simulink model "PubIfDecisionTOS_MDL"  (R2020b)
settings: configuration reference "DspaceConfig" (kept outside this file)
PostLoadFcn:
  | if any(exist('dsrtsu_mdlpostloadfcn', 'file') ~= 0), dsrtsu_mdlpostloadfcn('Execute', bdroot); end
InitFcn:
  | , if any(exist('dsmpb_private', 'file') ~= 0), dsmpb_private('dsmpb_mdlclblib', 'Init', bdroot); end,
undefined symbols (not defined in the file or in its folder): C_TOS_ACCEgoRAxletoFbumplength_m, C_TOS_ACCTargetFront_Flag, C_TOS_AEBJAPedObjDxThre_Val, C_TOS_AEBJAPedObjDyThre_Val, C_TOS_AEBJATargetSize_Val, C_TOS_AEBJAVehObjDxThre_Val, C_TOS_AEBJAVehObjDyThre_Val, C_TOS_AEBJuncPedTargetSize_Val, C_TOS_AEBLatObjDxThre_Val, C_TOS_AEBLatPedDyThre_Val, C_TOS_AEBLatTargetSize_Val, C_TOS_AEBLongTargetInEgoFront_Flag, C_TOS_axAbsGround_Parameter, C_TOS_CameraConfirmedFlag, C_TOS_CNsubjWidth, C_TOS_CurrentLaneCoreMinWidth_Val, C_TOS_CutInProb_Val_Zero, C_TOS_CutOutProb_Val_Zero, C_TOS_D2R_Val, C_TOS_DefaultValueObjectToCenterLine_dy, C_TOS_EgoCarWidth_Val, C_TOS_EgoDxRefPoint_m, C_TOS_EgoRAxletoFbumplength_m, C_TOS_HalfWidthVehicle_Con, C_TOS_HWA_CurrentLaneFlag, C_TOS_HWA_LeftLaneFlag, C_TOS_HWA_MovingDir_Vaild, C_TOS_HWA_MovState_Vaild, C_TOS_HWA_RightLaneFlag, C_TOS_LaneLineCourseErrorFront, C_TOS_LaneLineCourseErrorRear, C_TOS_MotorbikeDefaultWidth_m, C_TOS_NumberOfEffectiveTargets, C_TOS_Obj_Age_Val, C_TOS_Objdx_Constraint_Val, C_TOS_ObjectDefaultWidth_m, C_TOS_ObjInCurrentLane_Val, C_TOS_ObjInCurrentLaneValid, C_TOS_ObjInLeftLaneValid, C_TOS_ObjInRightLaneValid, C_TOS_ObjNotInCurrentLane_Val, C_TOS_ObjNotREElementType, C_TOS_ObjPredictDis_dy_ConstantVal_Zeros, C_TOS_ObjToCenterLine_ConstantVal_Zeros, C_TOS_OFMObjIDInvilad_Val, C_TOS_PIL_LatDisCons_Val_zero, C_TOS_PIL_ObjectCutInFlag_b, C_TOS_PIL_ObjectCutOutFlag_b, C_TOS_PIL_ObjLaneProb_al_Val, C_TOS_PP_ObjFusType_FC_Confirm_b, C_TOS_PP_ObjFusType_FC_FR_Confirm_b, C_TOS_PP_ObjFusType_FR_Confirm_b, C_TOS_RE_80BoolDefault_Val, C_TOS_RE_80Single181Default_Val, C_TOS_RE_80Single255Default_Val, C_TOS_RE_80Uint8Default_Val, C_TOS_RE_D2R, C_TOS_RE_D_180_Val, C_TOS_RE_InvalidObjectID_Val, C_TOS_RE_InvalidTargetChainDir_Val ... (+142)
libraries: simulink x1650, TOS_LIB x361, canfdmsglib x14
(part 65 of 69)

== stateflow chart PubIfDecisionTOS_MDL/TOS_20201112/TOS_2012080320/TOS/AEB/TOS_AEBJunct1105/AEBJunctionTargetInfor/TOS_AEBJunct ==
  (default) -> (junction 1) : {i=uint8(1);}
  (junction 1) -> (junction 40) [order 1] : [i<=C_TOS_AEBJATargetSize_Val]
  (junction 42) -> (junction 1) : {i=i+uint8(1);}
  (junction 1) -> (junction 60) [order 2]
  (junction 40) -> (junction 42) : {
      | TOS_AEBJuncTargetBus(i).FusionType= uint8(0);
      | TOS_AEBJuncTargetBus(i).ObjectID= uint8(0);
      | TOS_AEBJuncTargetBus(i).ObjectType= uint8(0);
      | TOS_AEBJuncTargetBus(i).ObjectTypeCameraConfirmed= false;
      | TOS_AEBJuncTargetBus(i).ObjectLength=single(0);
      | TOS_AEBJuncTargetBus(i).ObjectWidth= single(0);
      | TOS_AEBJuncTargetBus(i).ObjectHight= single(0);
      | TOS_AEBJuncTargetBus(i).ObjectYawAngle= single(0);
      | TOS_AEBJuncTargetBus(i).ObjectAzimuthAngle= single(0);
      | TOS_AEBJuncTargetBus(i).ObjectMovingState= uint8(0);
      | TOS_AEBJuncTargetBus(i).ObjectMovingOrientation=uint8(0);
      | TOS_AEBJuncTargetBus(i).dxFisrtDetection= single(0);
      | TOS_AEBJuncTargetBus(i).dyFisrtDetection= single(0);
      | TOS_AEBJuncTargetBus(i).dx= single(0);
      | TOS_AEBJuncTargetBus(i).dy= single(0);
      | TOS_AEBJuncTargetBus(i).dz= single(0);
      | TOS_AEBJuncTargetBus(i).vx= single(0);
      | TOS_AEBJuncTargetBus(i).vy= single(0);
      | TOS_AEBJuncTargetBus(i).ax= single(0);
      | TOS_AEBJuncTargetBus(i).ay= single(0);
      | TOS_AEBJuncTargetBus(i).dxVariance= single(0);
      | TOS_AEBJuncTargetBus(i).dyVariance= single(0);
      | TOS_AEBJuncTargetBus(i).vxVariance= single(0);
      | TOS_AEBJuncTargetBus(i).vyVariance= single(0);
      | TOS_AEBJuncTargetBus(i).axVariance= single(0);
      | TOS_AEBJuncTargetBus(i).ayVariance= single(0);
      | TOS_AEBJuncTargetBus(i).ObjectLengthVar= single(0);
      | TOS_AEBJuncTargetBus(i).ObjectWidthVar= single(0);
      | TOS_AEBJuncTargetBus(i).ObjectYawAngleVar= single(0);
      | TOS_AEBJuncTargetBus(i).ObjectTypeProb= single(0);
      | TOS_AEBJuncTargetBus(i).ObjectMovingStateProb= single(0);
      | TOS_AEBJuncTargetBus(i).ObjectMovingOrientationProb= single(0);
      | TOS_AEBJuncTargetBus(i).ObjectExistProb= single(0);
      | TOS_AEBJuncTargetBus(i).ObjectIsObstacleProb= single(0);
      | TOS_AEBJuncTargetBus(i).ObjectRCS= single(0);
      | TOS_AEBJuncTargetBus(i).ObjectMeasurementStatus= single(0);
      | TOS_AEBJuncTargetBus(i).ObjectLifeCycle= uint16(0);
      | TOS_AEBJuncTargetBus(i).ObjUpdate= false;
      | }
  (junction 60) -> (junction 53) : {i=uint8(1);
      | j=uint8(1);}
  (junction 53) -> (junction 62) [order 1] : [i<=C_TOS_AEBJATargetSize_Val]
  (junction 66) -> (junction 53) : {i=i+uint8(1);}
  (junction 53) -> (junction 46) [order 2]
  (junction 62) -> (junction 64)
  (junction 64) -> (junction 3) [order 1] : [TOS_AEBJATargetIndex(i)~=uint8(0)]
  (junction 64) -> (junction 66) [order 2]
  (junction 3) -> (junction 5) : {
      | TargetIndex = TOS_AEBJATargetIndex(i);
      | TOS_AEBJuncTargetBus(j).FusionType=OFM_SignalVerification.Object_Fus_Type(TargetIndex);
      | TOS_AEBJuncTargetBus(j).ObjectID=OFM_SignalVerification.Object_ID(TargetIndex);
      | TOS_AEBJuncTargetBus(j).ObjectType=AEBJuncTargetObjectType(i);
      | TOS_AEBJuncTargetBus(j).ObjectTypeCameraConfirmed=TOS_AddAttributes.PP_CamareConfirmSignalProcessing(TargetIndex);
      | TOS_AEBJuncTargetBus(j).ObjectLength=OFM_SignalVerification.Object_Length(TargetIndex);
      | TOS_AEBJuncTargetBus(j).ObjectWidth=OFM_SignalVerification.Object_Width(TargetIndex);
      | TOS_AEBJuncTargetBus(j).ObjectHight=OFM_SignalVerification.Object_Hight(TargetIndex);
      | TOS_AEBJuncTargetBus(j).ObjectYawAngle=OFM_SignalVerification.Object_HeadingAngle(TargetIndex);
      | TOS_AEBJuncTargetBus(j).ObjectAzimuthAngle=OFM_SignalVerification.Object_YawAngle(TargetIndex);
      | TOS_AEBJuncTargetBus(j).ObjectMovingState=TOS_AddAttributes.PP_MovingState_AEB_SignalProcessing(TargetIndex);
      | TOS_AEBJuncTargetBus(j).ObjectMovingOrientation=TOS_AddAttributes.PP_ObjMovingDirSignalProcessing(TargetIndex);
      | TOS_AEBJuncTargetBus(j).dxFisrtDetection=TOS_AddAttributes.PP_ObjFirstDetect_Dx(TargetIndex);
      | TOS_AEBJuncTargetBus(j).dyFisrtDetection=TOS_AddAttributes.PP_ObjFirstDetect_Dy(TargetIndex);
      | TOS_AEBJuncTargetBus(j).dx=OFM_SignalVerification.Object_DX(TargetIndex);
      | TOS_AEBJuncTargetBus(j).dy=OFM_SignalVerification.Object_DY(TargetIndex);
      | TOS_AEBJuncTargetBus(j).dz= single(0);
      | TOS_AEBJuncTargetBus(j).vx=OFM_SignalVerification.Object_VX(TargetIndex);
      | TOS_AEBJuncTargetBus(j).vy=OFM_SignalVerification.Object_VY(TargetIndex);
      | TOS_AEBJuncTargetBus(j).ax=OFM_SignalVerification.Object_AX(TargetIndex);
      | TOS_AEBJuncTargetBus(j).ay=OFM_SignalVerification.Object_AY(TargetIndex);
      | TOS_AEBJuncTargetBus(j).dxVariance=OFM_SignalVerification.Object_Std_DX(TargetIndex);
      | TOS_AEBJuncTargetBus(j).dyVariance=OFM_SignalVerification.Object_Std_DY(TargetIndex);
      | TOS_AEBJuncTargetBus(j).vxVariance=OFM_SignalVerification.Object_Std_VX(TargetIndex);
      | TOS_AEBJuncTargetBus(j).vyVariance=OFM_SignalVerification.Object_Std_VY(TargetIndex);
      | TOS_AEBJuncTargetBus(j).axVariance=OFM_SignalVerification.Object_Std_AX(TargetIndex);
      | TOS_AEBJuncTargetBus(j).ayVariance=OFM_SignalVerification.Object_Std_AY(TargetIndex);
      | TOS_AEBJuncTargetBus(j).ObjectLengthVar=OFM_SignalVerification.Object_Std_Length(TargetIndex);
      | TOS_AEBJuncTargetBus(j).ObjectWidthVar=OFM_SignalVerification.Object_Std_Width(TargetIndex);
      | TOS_AEBJuncTargetBus(j).ObjectYawAngleVar=OFM_SignalVerification.Object_Std_HeadingAngle(TargetIndex);
      | TOS_AEBJuncTargetBus(j).ObjectTypeProb=OFM_SignalVerification.Object_Type_Prob(TargetIndex);
      | TOS_AEBJuncTargetBus(j).ObjectMovingStateProb= single(0);
      | TOS_AEBJuncTargetBus(j).ObjectMovingOrientationProb= single(0);
      | TOS_AEBJuncTargetBus(j).ObjectExistProb=OFM_SignalVerification.Object_ExistProb(TargetIndex);
      | TOS_AEBJuncTargetBus(j).ObjectIsObstacleProb=OFM_SignalVerification.Object_ObstacleProb(TargetIndex);
      | TOS_AEBJuncTargetBus(j).ObjectRCS= single(0);
      | TOS_AEBJuncTargetBus(j).ObjectMeasurementStatus= single(0);
      | TOS_AEBJuncTargetBus(j).ObjectLifeCycle=OFM_SignalVerification.Object_Age(TargetIndex);
      | TOS_AEBJuncTargetBus(j).ObjUpdate= false;
      | j=j+uint8(1);
      | }
  (junction 5) -> (junction 66)
  data: TOS_AddAttributes input Bus: TOS_AddAttributes_BUS; OFM_SignalVerification input Bus: OFM_OBJ_BUS; AEBJuncTargetObjectType input uint8; TOS_AEBJATargetIndex input uint8; TOS_AEBJuncTargetBus output Bus: TOS_AEB_JAOBJ_BUS size=32 =0; C_TOS_AEBJATargetSize_Val parameter; TargetIndex local uint8 size=1; i local uint8 size=1; j local uint8 size=1

== matlab function PubIfDecisionTOS_MDL/TOS_20201112/TOS_2012080320/TOS/AEB/TOS_AEBJunct_20201208/AEBJuncTargetIndex/MATLAB Function ==
  data: Distance input; Object_Num input; ObjDisIndex output
function ObjDisIndex  = fcn(Distance,Object_Num)
ObjNum=80;
ObjDisIndex=uint8(zeros(ObjNum,1));
DxDy=Distance;
MidIndex=1:1:ObjNum;
for i=1:Object_Num
    ObjDisIndex(i)=MidIndex(i);
    t_dis=DxDy(i);
    if i<Object_Num-1
        for j=(i+1):Object_Num
            if DxDy(j)<t_dis
                temp_index=ObjDisIndex(i);
                temp_dis=t_dis;
                ObjDisIndex(i)=MidIndex(j);
                DxDy(i)=DxDy(j);
                t_dis=DxDy(j);
                MidIndex(j)=temp_index;
                DxDy(j)=temp_dis;
            end
            
            if DxDy(i) >= single(250)     
                ObjDisIndex(i)=uint8(0); 
            end           
   
        end
    else
        if i~=Object_Num
            if DxDy(Object_Num)<t_dis
                temp_index=ObjDisIndex(i);
                temp_dis=t_dis;
                ObjDisIndex(i)=MidIndex(Object_Num);
                DxDy(i)=DxDy(Object_Num);
                MidIndex(Object_Num)=temp_index;
                DxDy(Object_Num)=temp_dis;
            else
                MidIndex(Object_Num)=MidIndex(Object_Num);
                DxDy(Object_Num)=DxDy(Object_Num);
            end
            
            if DxDy(i) >= single(250)     
                ObjDisIndex(i)=uint8(0); 
            end       
            
        end
    end

end

== matlab function PubIfDecisionTOS_MDL/TOS_20201112/TOS_2012080320/TOS/AEB/TOS_AEBJunct_20201208/AEBJuncTargetIndex/MATLAB Function1 ==
  data: Object_Num input; Distance input; ObjDisIndex output
function ObjDisIndex  = fcn(Object_Num,Distance)
ObjNum=80;
ObjDisIndex=uint8(zeros(ObjNum,1));
DxDy=Distance;
MidIndex=1:1:ObjNum;
for i=1:Object_Num
    ObjDisIndex(i)=MidIndex(i);
    t_dis=DxDy(i);
    if i<Object_Num-1
        for j=(i+1):Object_Num
            if DxDy(j)<t_dis
                temp_index=ObjDisIndex(i);
                temp_dis=t_dis;
                ObjDisIndex(i)=MidIndex(j);
                DxDy(i)=DxDy(j);
                t_dis=DxDy(j);
                MidIndex(j)=temp_index;
                DxDy(j)=temp_dis;
            end
            
            if DxDy(i) >= single(250)     
                ObjDisIndex(i)=uint8(0); 
            end           
   
        end
    else
        if i~=Object_Num
            if DxDy(Object_Num)<t_dis
                temp_index=ObjDisIndex(i);
                temp_dis=t_dis;
                ObjDisIndex(i)=MidIndex(Object_Num);
                DxDy(i)=DxDy(Object_Num);
                MidIndex(Object_Num)=temp_index;
                DxDy(Object_Num)=temp_dis;
            else
                MidIndex(Object_Num)=MidIndex(Object_Num);
                DxDy(Object_Num)=DxDy(Object_Num);
            end
            
            if DxDy(i) >= single(250)     
                ObjDisIndex(i)=uint8(0); 
            end       
            
        end
    end

end

== stateflow chart PubIfDecisionTOS_MDL/TOS_20201112/TOS_2012080320/TOS/AEB/TOS_AEBJunct_20201208/AEBJunc_Object_Condition/AEBJA_TargetCondition/TOS_AEBJunc_TargetsCondition/AEBJunc_PedTargetCondition/Chart ==
  state AEBJuncSameTargetIDJudge [function]
    (default) -> (junction 70) : {
        | i = uint8(1);
        | AEBJunc_SameTarget = false;
        | }
    (junction 70) -> (junction 81) [order 1] : [i<=C_TOS_AEBJuncPedTargetSize_Val]
    (junction 86) -> (junction 70)
    (junction 70) -> (junction 83) [order 2]
    (junction 81) -> (junction 77)
    (junction 77) -> (junction 78) [order 1] : [AEBJunc_Target_ObjectID_K1(i) == Object_ID]
    (junction 77) -> (junction 74) [order 2] : %donothing
    (junction 78) -> (junction 72) : {
        | AEBJunc_SameTarget = true;
        | }
    (junction 72) -> (junction 74)
    (junction 74) -> (junction 86) : {i = i+1;}
  (default) -> (junction 1)
  (junction 1) -> (junction 3) [order 1] : [AEBJunc_TargetCondition == true]
  (junction 1) -> (junction 97) [order 2] : {
      | TOS_AEBJunc_TargetsDx = single(255);
      | }
  (junction 3) -> (junction 88) : {
      | AEBJuncSameTargetIDJudge();
      | }
  (junction 88) -> (junction 124) [order 1] : [AEBJunc_SameTarget == false]
  (junction 88) -> (junction 94) [order 2] : {
      | TOS_AEBJunc_TargetsDx = Object_Dx;
      | }
  (junction 124) -> (junction 114)
  (junction 114) -> (junction 117) [order 1] : [abs(Object_Vy) > P_TOS_AEBJuncTargetVyvThre_val ]
  (junction 114) -> (junction 118) [order 2] : {
      | TOS_AEBJunc_TargetsDx = single(255);
      | }
  (junction 117) -> (junction 112) : {
      | TOS_AEBJunc_TargetsDx = Object_Dx;
      | }
  (junction 112) -> (junction 118)
  (junction 118) -> (junction 125)
  (junction 94) -> (junction 97)
  (junction 125) -> (junction 94)
  (junction 97) -> (junction 100)
  data: AEBJunc_TargetCondition input boolean; Object_ID input uint8; psiDtOpt input single; AEBJunc_Target_ObjectID_K1 input uint8 size=32; Object_Vy input single; TOS_AEBJunc_TargetsDx output single size=1; Object_Dx input single; AEBJunc_SameTarget local boolean size=1 =false; P_TOS_AEBJuncTargetVyvThre_val parameter; P_TOS_AEBJuncTargetEgoYawRateThre_val parameter; C_TOS_AEBJuncPedTargetSize_Val parameter

== stateflow chart PubIfDecisionTOS_MDL/TOS_20201112/TOS_2012080320/TOS/AEB/TOS_AEBJunct_20201208/AEBJunc_Object_Condition/AEBJA_TargetCondition/TOS_AEBJunc_TargetsCondition/AEBJunc_VehTargetCondition/Chart ==
  state AEBJuncSameTargetIDJudge [function]
    (default) -> (junction 70) : {
        | i = uint8(1);
        | AEBJunc_SameTarget = false;
        | }
    (junction 70) -> (junction 81) [order 1] : [i<=C_TOS_AEBJuncPedTargetSize_Val]
    (junction 86) -> (junction 70)
    (junction 70) -> (junction 83) [order 2]
    (junction 81) -> (junction 77)
    (junction 77) -> (junction 78) [order 1] : [AEBJunc_Target_ObjectID_K1(i) == Object_ID]
    (junction 77) -> (junction 74) [order 2] : %donothing
    (junction 78) -> (junction 72) : {
        | AEBJunc_SameTarget = true;
        | }
    (junction 72) -> (junction 74)
    (junction 74) -> (junction 86) : {i = i+1;}
  (default) -> (junction 1)
  (junction 1) -> (junction 3) [order 1] : [AEBJunc_TargetCondition == true]
  (junction 1) -> (junction 97) [order 2] : {
      | TOS_AEBJunc_TargetsDx = single(255);
      | }
  (junction 3) -> (junction 88) : {
      | AEBJuncSameTargetIDJudge();
      | }
  (junction 88) -> (junction 124) [order 1] : [AEBJunc_SameTarget == false]
  (junction 88) -> (junction 94) [order 2] : {
      | TOS_AEBJunc_TargetsDx = Object_Dx;
      | }
  (junction 124) -> (junction 114)
  (junction 114) -> (junction 117) [order 1] : [abs(Object_Vy) > P_TOS_AEBJuncTargetVyvThre_val &&...
      | abs(psiDtOpt) < P_TOS_AEBJuncTargetEgoYawRateThre_val]
  (junction 114) -> (junction 118) [order 2] : {
      | TOS_AEBJunc_TargetsDx = single(255);
      | }
  (junction 117) -> (junction 112) : {
      | TOS_AEBJunc_TargetsDx = Object_Dx;
      | }
  (junction 112) -> (junction 118)
  (junction 118) -> (junction 125)
  (junction 94) -> (junction 97)
  (junction 125) -> (junction 94)
  (junction 97) -> (junction 100)
  data: AEBJunc_TargetCondition input boolean; Object_ID input uint8; psiDtOpt input single; AEBJunc_Target_ObjectID_K1 input uint8 size=32; Object_Vy input single; TOS_AEBJunc_TargetsDx output single size=1; Object_Dx input single; AEBJunc_SameTarget local boolean size=1 =false; P_TOS_AEBJuncTargetVyvThre_val parameter; P_TOS_AEBJuncTargetEgoYawRateThre_val parameter; C_TOS_AEBJuncPedTargetSize_Val parameter

== stateflow chart PubIfDecisionTOS_MDL/TOS_20201112/TOS_2012080320/TOS/AEB/TOS_AEBJunct_20201208/AEBJunc_Object_Condition1/AEBJA_TargetCondition/TOS_AEBJunc_TargetsCondition/AEBJunc_PedTargetCondition/Chart ==
  state AEBJuncSameTargetIDJudge [function]
    (default) -> (junction 70) : {
        | i = uint8(1);
        | AEBJunc_SameTarget = false;
        | }
    (junction 70) -> (junction 81) [order 1] : [i<=C_TOS_AEBJuncPedTargetSize_Val]
    (junction 86) -> (junction 70)
    (junction 70) -> (junction 83) [order 2]
    (junction 81) -> (junction 77)
    (junction 77) -> (junction 78) [order 1] : [AEBJunc_Target_ObjectID_K1(i) == Object_ID]
    (junction 77) -> (junction 74) [order 2] : %donothing
    (junction 78) -> (junction 72) : {
        | AEBJunc_SameTarget = true;
        | }
    (junction 72) -> (junction 74)
    (junction 74) -> (junction 86) : {i = i+1;}
  (default) -> (junction 1)
  (junction 1) -> (junction 3) [order 1] : [AEBJunc_TargetCondition == true]
  (junction 1) -> (junction 97) [order 2] : {
      | TOS_AEBJunc_TargetsDx = single(255);
      | }
  (junction 3) -> (junction 88) : {
      | AEBJuncSameTargetIDJudge();
      | }
  (junction 88) -> (junction 124) [order 1] : [AEBJunc_SameTarget == false]
  (junction 88) -> (junction 94) [order 2] : {
      | TOS_AEBJunc_TargetsDx = Object_Dx;
      | }
  (junction 124) -> (junction 114)
  (junction 114) -> (junction 117) [order 1] : [abs(Object_Vy) > P_TOS_AEBJuncTargetVyvThre_val &&...
      | abs(psiDtOpt) < P_TOS_AEBJuncTargetEgoYawRateThre_val]
  (junction 114) -> (junction 118) [order 2] : {
      | TOS_AEBJunc_TargetsDx = single(255);
      | }
  (junction 117) -> (junction 112) : {
      | TOS_AEBJunc_TargetsDx = Object_Dx;
      | }
  (junction 112) -> (junction 118)
  (junction 118) -> (junction 125)
  (junction 94) -> (junction 97)
  (junction 125) -> (junction 94)
  (junction 97) -> (junction 100)
  data: AEBJunc_TargetCondition input boolean; Object_ID input uint8; psiDtOpt input single; AEBJunc_Target_ObjectID_K1 input uint8 size=32; Object_Vy input single; TOS_AEBJunc_TargetsDx output single size=1; Object_Dx input single; AEBJunc_SameTarget local boolean size=1 =false; P_TOS_AEBJuncTargetVyvThre_val parameter; P_TOS_AEBJuncTargetEgoYawRateThre_val parameter; C_TOS_AEBJuncPedTargetSize_Val parameter

== stateflow chart PubIfDecisionTOS_MDL/TOS_20201112/TOS_2012080320/TOS/AEB/TOS_AEBJunct_20201208/AEBJunc_Object_Condition1/AEBJA_TargetCondition/TOS_AEBJunc_TargetsCondition/AEBJunc_VehTargetCondition/Chart ==
  state AEBJuncSameTargetIDJudge [function]
    (default) -> (junction 70) : {
        | i = uint8(1);
        | AEBJunc_SameTarget = false;
        | }
    (junction 70) -> (junction 81) [order 1] : [i<=C_TOS_AEBJuncPedTargetSize_Val]
    (junction 86) -> (junction 70)
    (junction 70) -> (junction 83) [order 2]
    (junction 81) -> (junction 77)
    (junction 77) -> (junction 78) [order 1] : [AEBJunc_Target_ObjectID_K1(i) == Object_ID]
    (junction 77) -> (junction 74) [order 2] : %donothing
    (junction 78) -> (junction 72) : {
        | AEBJunc_SameTarget = true;
        | }
    (junction 72) -> (junction 74)
    (junction 74) -> (junction 86) : {i = i+1;}
  (default) -> (junction 1)
  (junction 1) -> (junction 3) [order 1] : [AEBJunc_TargetCondition == true]
  (junction 1) -> (junction 97) [order 2] : {
      | TOS_AEBJunc_TargetsDx = single(255);
      | }
  (junction 3) -> (junction 88) : {
      | AEBJuncSameTargetIDJudge();
      | }
  (junction 88) -> (junction 124) [order 1] : [AEBJunc_SameTarget == false]
  (junction 88) -> (junction 94) [order 2] : {
      | TOS_AEBJunc_TargetsDx = Object_Dx;
      | }
  (junction 124) -> (junction 114)
  (junction 114) -> (junction 117) [order 1] : [abs(Object_Vy) > P_TOS_AEBJuncTargetVyvThre_val &&...
      | abs(psiDtOpt) < P_TOS_AEBJuncTargetEgoYawRateThre_val]
  (junction 114) -> (junction 118) [order 2] : {
      | TOS_AEBJunc_TargetsDx = single(255);
      | }
  (junction 117) -> (junction 112) : {
      | TOS_AEBJunc_TargetsDx = Object_Dx;
      | }
  (junction 112) -> (junction 118)
  (junction 118) -> (junction 125)
  (junction 94) -> (junction 97)
  (junction 125) -> (junction 94)
  (junction 97) -> (junction 100)
  data: AEBJunc_TargetCondition input boolean; Object_ID input uint8; psiDtOpt input single; AEBJunc_Target_ObjectID_K1 input uint8 size=32; Object_Vy input single; TOS_AEBJunc_TargetsDx output single size=1; Object_Dx input single; AEBJunc_SameTarget local boolean size=1 =false; P_TOS_AEBJuncTargetVyvThre_val parameter; P_TOS_AEBJuncTargetEgoYawRateThre_val parameter; C_TOS_AEBJuncPedTargetSize_Val parameter

== stateflow chart PubIfDecisionTOS_MDL/TOS_20201112/TOS_2012080320/PP1128/AAT-AdditionalAttributes/RoadEdge/RE_2020_12_07/RoadEdge_V2/RoadEdgeElementType/Chart ==
  state EdgeElementCounter [function]
    (default) -> (junction 24)
    (junction 24) -> (junction 37) [order 1] : [EdgeElementID(i) ~= uint8(0)]
    (junction 24) -> (junction 39) [order 2] : %donothing
    (junction 37) -> (junction 41) : {
        | EdgeElementCount(i) = EdgeElementCount(i)+uint8(1);
        | }
    (junction 41) -> (junction 39)
    (junction 39) -> (junction 82)
    (junction 82) -> (junction 84) [order 1] : [EdgeElementID(i) == uint8(0)]
    (junction 82) -> (junction 88) [order 2] : {
        | NotEdgeElementCount(i) = uint8(0);
        | }
    (junction 84) -> (junction 86) : {
        | NotEdgeElementCount(i) = NotEdgeElementCount(i)+uint8(1);
        | }
    (junction 86) -> (junction 88)
    (junction 88) -> (junction 43)
    (junction 43) -> (junction 46) [order 1] : [EdgeElementCount(i) >= uint8(255)]
    (junction 43) -> (junction 48) [order 2] : %donothing
    (junction 46) -> (junction 50) : {
        | EdgeElementCount(i) = uint8(255);
        | }
    (junction 50) -> (junction 48)
    (junction 48) -> (junction 53)
    (junction 53) -> (junction 91) [order 1] : [NotEdgeElementCount(i) >= uint8(255)]
    (junction 53) -> (junction 95) [order 2]
    (junction 91) -> (junction 93) : {
        | NotEdgeElementCount(i) = uint8(255);
        | }
    (junction 93) -> (junction 95)
    (junction 95) -> (junction 98)
  state FinalConfirm [function]
    state RE_Object_FR_Other = FusType(ObjectFusType) [function]
    (default) -> (junction 27)
    (junction 27) -> (junction 64) [order 1] : [RE_EdgeElementID_K1(i) ~= uint8(0)&&...
        | EdgeElementID(i) == uint8(0)]
    (junction 27) -> (junction 57) [order 2] : {
        | RE_EdgeElementID(i) = EdgeElementID(i);
        | RE_EdgeElementType(i) = EdgeElementType(i);
        | }
    (junction 64) -> (junction 66) : {
        | RE_Object_FR_Other = FusType(Object_FusType(i));
        | }
    (junction 66) -> (junction 55) [order 1] : [EdgeElementCount(i) >= uint8(10)&&...
        | Object_Age(i) >=uint8(10)&&...
        | Object_MovingState(i) == OFM_OBJ_MOVINGSTATE_E.STATIONARY&&...
        | RE_Object_FR_Other == true]
        | %连续选中1s、目标连续存在1s、目标静止、仅雷达探测
    (junction 66) -> (junction 71) [order 2] : {
        | RE_EdgeElementID(i) = EdgeElementID(i);
        | RE_EdgeElementType(i) = EdgeElementType(i);
        | }
    (junction 55) -> (junction 59) : {
        | RE_EdgeElementID(i) = RE_EdgeElementID_K1(i);
        | RE_EdgeElementType(i) = RE_EdgeElementType_K1(i);
        | }
    (junction 59) -> (junction 71)
    (junction 71) -> (junction 57)
    (junction 57) -> (junction 62)
    (junction 62) -> (junction 100) [order 1] : [NotEdgeElementCount(i) > EdgeElementCount(i)||...
        | NotEdgeElementCount(i) > uint8(40)]
        | %延时成为边界元素的时间，最多延时2s
    (junction 62) -> (junction 102) [order 2] : %donothing
    (junction 100) -> (junction 106) : {
        | RE_EdgeElementID(i) = EdgeElementID(i);
        | RE_EdgeElementType(i) = EdgeElementType(i);
        | }
    (junction 106) -> (junction 102)
    (junction 102) -> (junction 104)
  (default) -> (junction 6) : {
      | i = uint8(1);
      | }
  (junction 6) -> (junction 30) [order 1] : [i<=uint8(80)]
  (junction 34) -> (junction 6) : {
      | i= i+uint8(1);
      | }
  (junction 6) -> (junction 12) [order 2]
  (junction 30) -> (junction 31)
  (junction 31) -> (junction 8) [order 1] : [Object_ID(i) ~= C_TOS_RE_InvalidObjectID_Val]
  (junction 31) -> (junction 34) [order 2] : {
      | EdgeElementCount(i) = uint8(0);
      | RE_EdgeElementType(i) = uint8(0);
      | RE_EdgeElementID(i) = uint8(0);
      | }
  (junction 8) -> (junction 21) : {
      | EdgeElementCounter();
      | }
  (junction 21) -> (junction 14) : {
      | FinalConfirm();
      | }
  (junction 14) -> (junction 34)
  (junction 12) -> (junction 17)
  data: ObjectFusType function_input uint8 size=1; RE_Object_FR_Other function_output; EdgeElementType input uint8 size=80; EdgeElementID input uint8 size=80; RE_EdgeElementType output uint8 size=80; RE_EdgeElementID output uint8 size=80; Object_Age input uint16 size=80; Object_ID input uint8 size=80; Object_MovingState input Enum: OFM_OBJ_MOVINGSTATE_E size=80; Object_FusType input uint8 size=80; RE_EdgeElementType_K1 input uint8 size=80; RE_EdgeElementID_K1 input uint8 size=80; i local uint8 size=1; EdgeElementCount local uint8 size=80 [..255] =C_TOS_RE_80Uint8Default_Val; NotEdgeElementCount local uint8 size=80 =C_TOS_RE_80Uint8Default_Val; C_TOS_RE_InvalidObjectID_Val parameter; RE_Object_FR_Other local boolean size=1; Object_FusType_i local uint8 size=1

== stateflow chart PubIfDecisionTOS_MDL/TOS_20201112/TOS_2012080320/PP1128/AAT-AdditionalAttributes/RoadEdge/RE_2020_12_07/RoadEdge_V2/RoadEdgeElementType/For Each Subsystem/StateDelayAbortion ==
  state NormalState
    en:
    stateOut = state;
    CNTimeCounterMAX = 256;
    du:
    stateOut = state;
  state CounterState
    en:
    timeSinceLastState = 0;
    state_K1 = stateK1;
    du:
    timeSinceLastState +=  Ts;
    CounterStateFunc();
  state CounterStateFunc [function]
    (default) -> (junction 70)
    (junction 70) -> (junction 62) [order 1] : [timeSinceLastState > CNTimeCounterMAX]
    (junction 70) -> (junction 69) [order 2] : %do nothing
    (junction 62) -> (junction 61) : {
        | 	timeSinceLastState = CNTimeCounterMAX;
        | }
    (junction 61) -> (junction 69)
    (junction 69) -> (junction 68)
    (junction 68) -> (junction 60) [order 1] : [timeSinceLastState <= stateProlongationTime]
    (junction 68) -> (junction 66) [order 2] : {
        | 	stateOut = state;
        | }
    (junction 60) -> (junction 67) : {
        | 	stateOut = state_K1;
        | }
    (junction 67) -> (junction 66)
    (junction 66) -> (junction 56)
  (default) -> NormalState
  NormalState -> CounterState : [stateK1 != uint8(0) &&...
      | state == uint8(0)]
  CounterState -> NormalState : [timeSinceLastState > stateProlongationTime]
  data: state input; stateK1 input; stateProlongationTime input; timeSinceLastState output double; stateOut output uint8; Ts input; CNTimeCounterMAX local double; state_K1 local uint8

== stateflow chart PubIfDecisionTOS_MDL/TOS_20201112/TOS_2012080320/PP1128/AAT-AdditionalAttributes/RoadEdge/RE_2020_12_07/RoadEdge_V2/RoadEdgeElementType/For Each Subsystem1/StateDelayAbortion ==
  state NormalState
    en:
    stateOut = state;
    CNTimeCounterMAX = 256;
    du:
    stateOut = state;
  state CounterState
    en:
    timeSinceLastState = 0;
    state_K1 = stateK1;
    du:
    timeSinceLastState +=  Ts;
    CounterStateFunc();
  state CounterStateFunc [function]
    (default) -> (junction 70)
    (junction 70) -> (junction 62) [order 1] : [timeSinceLastState > CNTimeCounterMAX]
    (junction 70) -> (junction 69) [order 2] : %do nothing
    (junction 62) -> (junction 61) : {
        | 	timeSinceLastState = CNTimeCounterMAX;
        | }
    (junction 61) -> (junction 69)
    (junction 69) -> (junction 68)
    (junction 68) -> (junction 60) [order 1] : [timeSinceLastState <= stateProlongationTime]
    (junction 68) -> (junction 66) [order 2] : {
        | 	stateOut = state;
        | }
    (junction 60) -> (junction 67) : {
        | 	stateOut = state_K1;
        | }
    (junction 67) -> (junction 66)
    (junction 66) -> (junction 56)
  (default) -> NormalState
  NormalState -> CounterState : [stateK1 != uint8(0) &&...
      | state == uint8(0)]
  CounterState -> NormalState : [timeSinceLastState > stateProlongationTime]
  data: state input; stateK1 input; stateProlongationTime input; timeSinceLastState output double; stateOut output uint8; Ts input; CNTimeCounterMAX local double; state_K1 local uint8

== stateflow chart PubIfDecisionTOS_MDL/TOS_20201112/TOS_2012080320/PP1128/AAT-AdditionalAttributes/RoadEdge/RE_2020_12_07/RoadEdge_V2/RoadEdgeGroupChain/EgoLeft_RoadEdgeGroupChain ==
  state TargetChain_ObjDxDyAverageCal [function]
    state TCObjDxAve_Cal [function]
      (default) -> (junction 542) : {
          | j=uint8(1);
          | OFM_Object_Index = RE_StillObjectSortIndex[i] - uint8(1);
          | Start_Index_1 = OFM_Object_Index;
          | TargetChain_ObjectDx_1 = C_TOS_RE_80Single255Default_Val;
          | TargetChain_ObjectDx_2 = C_TOS_RE_80Single255Default_Val;
          | TargetChain_ObjectDx_3 = C_TOS_RE_80Single255Default_Val;
          | TargetChain_ObjectDx_4 = C_TOS_RE_80Single255Default_Val;
          | Sum_TargetChain_ObjectDx_1 = single(0);
          | Sum_TargetChain_ObjectDx_2 = single(0);
          | Sum_TargetChain_ObjectDx_3 = single(0);
          | Sum_TargetChain_ObjectDx_4 = single(0);
          | }
      (junction 542) -> (junction 543) [order 1] : [ j <= TargetChainElementNum[i] ]
      (junction 553) -> (junction 542) : {
          | j=j+uint8(1);
          | }
      (junction 542) -> (junction 552) [order 2]
      (junction 543) -> (junction 544) : {
          | StartDx_1 = ObjectDx[Start_Index_1];
          | TargetChain_ObjectDx_1[j] = ObjectDx[OFM_Object_Index];
          | }
      (junction 544) -> (junction 545) [order 1] : [TargetChain_ObjectDx_1[j] >= StartDx_1 &&...
          | abs(StartDx_1 - TargetChain_ObjectDx_1[j]) <= single(50)]
      (junction 544) -> (junction 546) [order 2] : {
          | Start_Index_2 = RE_StillObjectSortIndex[i+TargetChain_ObjectNum_1] - uint8(1);
          | StartDx_2 = ObjectDx[Start_Index_2];
          | TargetChain_ObjectDx_2[j] = ObjectDx[OFM_Object_Index];
          | }
      (junction 545) -> (junction 557) : {
          | TargetChainPart[i+j - uint8(1)] = uint8(1);
          | TargetChain_ObjectDx_1[j] = ObjectDx[OFM_Object_Index];
          | Sum_TargetChain_ObjectDx_1 = Sum_TargetChain_ObjectDx_1 + TargetChain_ObjectDx_1[j];
          | TargetChain_ObjectNum_1 = j;
          | OFM_Object_Index = RE_StillObjectSortIndex[i+j] - uint8(1);%索引值变到目标链上的下一个目标
          | }
      (junction 546) -> (junction 547) [order 1] : [TargetChain_ObjectDx_2[j] >= StartDx_2 &&...
          | abs(StartDx_2 - TargetChain_ObjectDx_2[j]) <= single(50)]
      (junction 546) -> (junction 548) [order 2] : {
          | Start_Index_3 = RE_StillObjectSortIndex[i + TargetChain_ObjectNum_1 + TargetChain_ObjectNum_2]  - uint8(1);
          | StartDx_3 = ObjectDx[Start_Index_3];
          | TargetChain_ObjectDx_3[j] = ObjectDx[OFM_Object_Index];
          | }
      (junction 547) -> (junction 556) : {
          | TargetChainPart[i+j - uint8(1)] = uint8(2);
          | TargetChain_ObjectDx_2[j] = ObjectDx[OFM_Object_Index];
          | Sum_TargetChain_ObjectDx_2 = Sum_TargetChain_ObjectDx_2 + TargetChain_ObjectDx_2[j];
          |  TargetChain_ObjectNum_2 = j - TargetChain_ObjectNum_1;
          | OFM_Object_Index = RE_StillObjectSortIndex[i+j] - uint8(1);%索引值变到目标链上的下一个目标
          | }
      (junction 548) -> (junction 549) [order 1] : [TargetChain_ObjectDx_3[j] >= StartDx_3 &&...
          | abs(StartDx_3 - TargetChain_ObjectDx_3[j]) <= single(50)]
      (junction 548) -> (junction 550) [order 2] : {
          | Start_Index_4 = RE_StillObjectSortIndex[i + TargetChain_ObjectNum_1 + TargetChain_ObjectNum_2 + TargetChain_ObjectNum_3]  - uint8(1);
          | StartDx_4 = ObjectDx[Start_Index_4];
          | TargetChain_ObjectDx_4[j] = ObjectDx[OFM_Object_Index];
          | }
      (junction 549) -> (junction 555) : {
          | TargetChainPart[i+j - uint8(1)] = uint8(3);
          | TargetChain_ObjectDx_3[j] = ObjectDx[OFM_Object_Index];
          | Sum_TargetChain_ObjectDx_3 = Sum_TargetChain_ObjectDx_3 + TargetChain_ObjectDx_3[j];
          |  TargetChain_ObjectNum_3 = j - TargetChain_ObjectNum_2 - TargetChain_ObjectNum_1 ;
          | OFM_Object_Index = RE_StillObjectSortIndex[i+j] - uint8(1);%索引值变到目标链上的下一个目标
          | }
      (junction 550) -> (junction 551) [order 1] : [TargetChain_ObjectDx_4[j] >= StartDx_4 &&...
          | abs(StartDx_4 - TargetChain_ObjectDx_4[j]) <= single(50)]
      (junction 550) -> (junction 553) [order 2] : {
          | TargetChainPart[i+j - uint8(1)]= uint8(0);
          | TargetChain_ObjectDx_Average_1 = single(255);
          | TargetChain_ObjectDx_Average_2 = single(255);
          | TargetChain_ObjectDx_Average_3 = single(255);
          | TargetChain_ObjectDx_Average_4 = single(255);
          | %同一目标链上的所有元素的Dx平均值，Dx平均值
          | }
      (junction 551) -> (junction 554) : {
          | TargetChainPart[i+j - uint8(1)]= uint8(4);
          | TargetChain_ObjectDx_4[j] = ObjectDx[OFM_Object_Index];
          | Sum_TargetChain_ObjectDx_4 = Sum_TargetChain_ObjectDx_4 + TargetChain_ObjectDx_4[j];
          | TargetChain_ObjectNum_4 = j - TargetChain_ObjectNum_3 - TargetChain_ObjectNum_2 - TargetChain_ObjectNum_1 ;
          | OFM_Object_Index = RE_StillObjectSortIndex[i+j] - uint8(1);%索引值变到目标链上的下一个目标
          | }
      (junction 554) -> (junction 553)
      (junction 555) -> (junction 554)
      (junction 556) -> (junction 555)
      (junction 557) -> (junction 556)
      (junction 552) -> (junction 558) : {
          | TargetChain_ObjectDx_Average_1 = Sum_TargetChain_ObjectDx_1/TargetChain_ObjectNum_1;
          | TargetChain_ObjectDx_Average_2 = Sum_TargetChain_ObjectDx_2/TargetChain_ObjectNum_2;
          | TargetChain_ObjectDx_Average_3 = Sum_TargetChain_ObjectDx_3/TargetChain_ObjectNum_3;
          | TargetChain_ObjectDx_Average_4 = Sum_TargetChain_ObjectDx_4/TargetChain_ObjectNum_4;
          | %同一目标链上的所有元素的Dx平均值，Dx平均值
          | }
    state TCObjDyAve_Cal [function]
      (default) -> (junction 481) : {
          | j=uint8(1);
          | OFM_Object_Index = RE_StillObjectSortIndex[i] - uint8(1);
          | Sum_TargetChain_ObjectDy = single(0);
          | }
      (junction 481) -> (junction 473) [order 1] : [ j <= TargetChainElementNum[i] ]
      (junction 475) -> (junction 481) : {
          | j=j+uint8(1);
          | }
      (junction 481) -> (junction 470) [order 2]
      (junction 473) -> (junction 475) : {
          | TargetChain_ObjectDy[j] = ObjectDy[OFM_Object_Index];
          | Sum_TargetChain_ObjectDy = Sum_TargetChain_ObjectDy + TargetChain_ObjectDy[j];
          | OFM_Object_Index = RE_StillObjectSortIndex[i+j] - uint8(1);
          | }
      (junction 470) -> (junction 480) : {
          | TargetChain_ObjectDy_Average[i] = Sum_TargetChain_ObjectDy/TargetChainElementNum[i];
          | %同一目标链上的所有元素的Dy平均值
          | }
    state TargetChain_ObjectDx_Average [function]
      state TargetChainPart4_DxAve [function]
        (default) -> (junction 626)
        (junction 626) -> (junction 635) [order 1] : [TargetChain_ObjectNum_4 <=uint8(2)]
        (junction 626) -> (junction 630) [order 2] : {
            | TargetChain_ObjectDx_Average[i] = TargetChain_ObjectDx_Average_4;
            | }
        (junction 635) -> (junction 633) : {
            | TargetChain_ObjectDx_Average[i] = (TargetChain_ObjectDx_Average_4+TargetChain_ObjectDx_Average_3)/2;
            | }
        (junction 633) -> (junction 630)
        (junction 630) -> (junction 636)
      state TargetChainPart3_DxAve [function]
        (default) -> (junction 655)
        (junction 655) -> (junction 653) [order 1] : [TargetChain_ObjectNum_3 <=uint8(2)]
        (junction 655) -> (junction 643) [order 2] : {
            | TargetChain_ObjectDx_Average[i] = TargetChain_ObjectDx_Average_3;
            | }
        (junction 653) -> (junction 644) : {
            | TargetChain_ObjectDx_Average[i] = (TargetChain_ObjectDx_Average_3+TargetChain_ObjectDx_Average_2)/2;
            | }
        (junction 644) -> (junction 643)
        (junction 643) -> (junction 645)
      state TargetChainPart2_DxAve [function]
        (default) -> (junction 672)
        (junction 672) -> (junction 674) [order 1] : [TargetChain_ObjectNum_2 <=uint8(2)]
        (junction 672) -> (junction 662) [order 2] : {
            | TargetChain_ObjectDx_Average[i] = TargetChain_ObjectDx_Average_2;
            | }
        (junction 674) -> (junction 663) : {
            | TargetChain_ObjectDx_Average[i] = (TargetChain_ObjectDx_Average_2+TargetChain_ObjectDx_Average_1)/2;
            | }
        (junction 663) -> (junction 662)
        (junction 662) -> (junction 664)
      (default) -> (junction 483)
      (junction 483) -> (junction 485) [order 1] : [TargetChainPart[i] == uint8(1)]
      (junction 483) -> (junction 491) [order 2]
      (junction 485) -> (junction 489) : {
          | TargetChain_ObjectDx_Average[i] = TargetChain_ObjectDx_Average_1;
          | }
      (junction 491) -> (junction 495) [order 1] : [TargetChainPart[i] == uint8(2)]
      (junction 491) -> (junction 493) [order 2]
      (junction 495) -> (junction 509) : {
          | TargetChainPart2_DxAve();
          | }
      (junction 493) -> (junction 497) [order 1] : [TargetChainPart[i] == uint8(3)]
      (junction 493) -> (junction 501) [order 2]
      (junction 497) -> (junction 499) : {
          | TargetChainPart3_DxAve();
          | }
      (junction 501) -> (junction 503) [order 1] : [TargetChainPart[i] == uint8(4)]
      (junction 501) -> (junction 487) [order 2] : {
          | TargetChain_ObjectDx_Average[i] = single(255);
          | }
      (junction 503) -> (junction 637) : {
          | TargetChainPart4_DxAve();
          | }
      (junction 637) -> (junction 487)
      (junction 499) -> (junction 637)
      (junction 509) -> (junction 499)
      (junction 489) -> (junction 509)
      (junction 487) -> (junction 513)
    (default) -> (junction 55)
    (junction 55) -> (junction 56) [order 1] : [ TargetChainStartIndex[i] != uint8(0)&&i == (TargetChainStartIndex[i]-uint8(1)) ]
        | %  i  目标 是目标链起始元素
    (junction 56) -> (junction 381) : {
        | TCObjDxAve_Cal();
        | TCObjDyAve_Cal();
        | }
    (junction 55) -> (junction 64) [order 2]
    (junction 64) -> (junction 66) [order 1] : [ (TargetChainStartIndex[i] != uint8(0))&&(i > (TargetChainStartIndex[i]-uint8(1)) )]
        | %目标i是目标链的剩余元素
    (junction 64) -> (junction 58) [order 2] : {
        | TargetChain_ObjectDx_Average[i] = single(255);
        | TargetChain_ObjectDy_Average[i] = single(255);
        | }
    (junction 66) -> (junction 68) : {
        | TargetChain_ObjectDx_Average();
        | TargetChain_ObjectDy_Average[i] = TargetChain_ObjectDy_Average[i - uint8(1)];
        | %同一目标链上的所有元素的Dx平均值，Dy平均值
        | }
    (junction 381) -> (junction 34) : {
        | TargetChain_ObjectDx_Average[i] = TargetChain_ObjectDx_Average_1;
        | }
    (junction 68) -> (junction 58)
    (junction 34) -> (junction 68)
    (junction 58) -> (junction 62)
  state RoadEdgeGroupChainJudge [function]
    (default) -> (junction 43) : {
        | OFM_Object_Index = RE_StillObjectSortIndex[i] - uint8(1);
        | }
    (junction 43) -> (junction 52) [order 1] : [abs(ObjectDx[OFM_Object_Index] - TargetChain_ObjectDx_Average[i]) < P_TOS_RE_RoadEdgeGroupDxThre_Val]
    (junction 43) -> (junction 47) [order 2] : {
        | REGroupChainFlag[i] =false;
        | }
    (junction 52) -> (junction 74)
    (junction 74) -> (junction 76) [order 1] : [Ego_Velocity > P_TOS_RE_RoadEdgeGroupEgoVxvThre_Val&&...
        | (abs(ObjectDy[OFM_Object_Index] - TargetChain_ObjectDy_Average[i]) < P_TOS_RE_RoadEdgeGroupDy_HighSpeedThre_Val)]
    (junction 74) -> (junction 78) [order 2]
    (junction 76) -> (junction 84) : {
        | REGroupChainFlag[i] = true;
        | }
    (junction 78) -> (junction 80) [order 1] : [Ego_Velocity <= P_TOS_RE_RoadEdgeGroupEgoVxvThre_Val &&...
        | (abs(ObjectDy[OFM_Object_Index] - TargetChain_ObjectDy_Average[i]) < P_TOS_RE_RoadEdgeGroupDy_LowSpeedThre_Val)]
    (junction 78) -> (junction 86) [order 2] : {
        | REGroupChainFlag[i] =false;
        | }
    (junction 80) -> (junction 82) : {
        | REGroupChainFlag[i] = true;
        | }
    (junction 86) -> (junction 47)
    (junction 82) -> (junction 86)
    (junction 84) -> (junction 82)
    (junction 47) -> (junction 93)
  state REGroupChainNumCal [function]
    note: 计算连续满足条件的边界组链的元素个数
        | 给边界组链中元素编号
    note: 3个目标组成一条链目标连；
        | 计算得到目标链的起始目标在Dx排序中的Index+1；
    (default) -> (junction 204)
    (junction 204) -> (junction 205) [order 1] : [i == uint8(0)]
        | %从每个目标链的第一个元素开始计数
    (junction 204) -> (junction 581) [order 2]
    (junction 205) -> (junction 211)
    (junction 581) -> (junction 584) [order 1] : [i > uint8(0)&&...
        | TargetChainStartIndex[i] !=uint8(0)&&...
        | TargetChainStartIndex[i-uint8(1)] !=uint8(0)&&...
        | TargetChainStartIndex[i] != TargetChainStartIndex[i - uint8(1)]]
        | %从每个目标链的第一个元素开始计数
    (junction 581) -> (junction 122) [order 2]
    (junction 584) -> (junction 589)
    (junction 589) -> (junction 598) [order 1] : [REGroupChainFlag[i] == true]
    (junction 211) -> (junction 213) [order 1] : [REGroupChainFlag[i] == true]
    (junction 122) -> (junction 123) [order 1] : [REGroupChainFlag[i] == true]
    (junction 589) -> (junction 597) [order 2] : {
        | GroupChainElementCounter[i] = uint8(0);
        | }
    (junction 598) -> (junction 594) : {
        | GroupChainElementCounter[i] = uint8(1);
        | }
    (junction 211) -> (junction 208) [order 2] : {
        | GroupChainElementCounter[i] = uint8(0);
        | }
    (junction 213) -> (junction 215) : {
        | GroupChainElementCounter[i] = uint8(1);
        | }
    (junction 122) -> (junction 124) [order 2] : {
        | GroupChainElementCounter[i] = uint8(0);
        | }
    (junction 123) -> (junction 125) : {
        | GroupChainElementCounter[i] = GroupChainElementCounter[i-uint8(1)] + uint8(1);
        | }
    (junction 125) -> (junction 124)
    (junction 597) -> (junction 125)
    (junction 594) -> (junction 597)
    (junction 208) -> (junction 594)
    (junction 215) -> (junction 208)
    (junction 124) -> (junction 126)
    (junction 126) -> (junction 127) [order 1] : [GroupChainElementCounter[i] == uint8(3)]
        | %连续3个目标符合条件时，组成边界组链；
    (junction 126) -> (junction 128) [order 2]
    (junction 127) -> (junction 132) : {
        | GroupChainStartIndex[i - uint8(2)] = i - uint8(1);
        | GroupChainStartIndex[i - uint8(1)] = i - uint8(1);
        | GroupChainStartIndex[i] = i - uint8(1) ;
        | %GroupChainElementCounter[i - uint8(2)] = uint8(1);
        | %GroupChainElementCounter[i - uint8(1)] = uint8(2);
        | %边界组链元素起始目标Index从1开始计数
        | }
    (junction 128) -> (junction 129) [order 1] : [GroupChainElementCounter[i]  > uint8(3)]
    (junction 128) -> (junction 130) [order 2] : {
        | GroupChainStartIndex[i] = uint8(0);
        | %GroupChainElementCounter[i] = uint8(0);
        | }
    (junction 129) -> (junction 131) : {
        | GroupChainStartIndex[i] = GroupChainStartIndex[i - uint8(1)] ;
        | %边界组链元素i序号不变
        | }
    (junction 131) -> (junction 130)
    (junction 132) -> (junction 131)
    (junction 130) -> (junction 226)
  (default) -> (junction 2) : {
      | i = uint8(0);
      | TargetChainPart = C_TOS_RE_80Uint8Default_Val;
      | TargetChain_ObjectDx_Average = C_TOS_RE_80Single255Default_Val;
      | TargetChain_ObjectDy_Average = C_TOS_RE_80Single255Default_Val;
      | REGroupChainFlag = C_TOS_RE_80BoolDefault_Val;
      | GroupChainElementCounter = C_TOS_RE_80Uint8Default_Val;
      | GroupChainStartIndex = C_TOS_RE_80Uint8Default_Val;
      | }
      | %从第1个目标开始
  (junction 2) -> (junction 3) [order 1] : [RE_StillObjectSortIndex[i] ~= C_TOS_StillObjSortInvalidIndex_Val&&...
      | i <= uint8(79)]
  (junction 118) -> (junction 2) : {
      | i = i+uint8(1);
      | }
  (junction 2) -> (junction 5) [order 2]
  (junction 3) -> (junction 38) : {
      | TargetChain_ObjDxDyAverageCal();
      | }
  (junction 38) -> (junction 7) : {
      | RoadEdgeGroupChainJudge();
      | }
  (junction 7) -> (junction 118) : {
      | REGroupChainNumCal();
      | }
  (junction 5) -> (junction 10)
  data: GroupChainElementCounter output uint8 size=80; GroupChainStartIndex output uint8 size=80; C_TOS_StillObjSortInvalidIndex_Val parameter; ObjectDx input size=80; ObjectDy input size=80; P_TOS_RE_RoadEdgeGroupDxThre_Val parameter; RE_StillObjectSortIndex input size=80; TargetChainElementNum input size=80; TargetChainStartIndex input size=80; REGroupChainFlag output uint8 size=80; OFM_Object_Index local uint8 size=1; TargetChain_ObjectDy local single size=80; i local uint8 size=1; j local uint8 size=1; Ego_Velocity input size=1; P_TOS_RE_RoadEdgeGroupDy_HighSpeedThre_Val parameter; P_TOS_RE_RoadEdgeGroupDy_LowSpeedThre_Val parameter; P_TOS_RE_RoadEdgeGroupEgoVxvThre_Val parameter; Sum_TargetChain_ObjectDy local single size=1; RE_TargetChainIndex input uint8 size=80; C_TOS_RE_80Single255Default_Val parameter; C_TOS_RE_80BoolDefault_Val parameter; C_TOS_RE_80Uint8Default_Val parameter; StartDx_1 local single size=1 =255; StartDx_2 local single size=1 =255; StartDx_3 local single size=1 =255; StartDx_4 local single size=1 =255; Start_Index_1 local uint8 size=1 =0; Start_Index_2 local uint8 size=1 =0; Start_Index_3 local uint8 size=1 =0; Start_Index_4 local uint8 size=1 =0; Sum_TargetChain_ObjectDx_1 local single size=1 =0; Sum_TargetChain_ObjectDx_2 local single size=1 =0; Sum_TargetChain_ObjectDx_3 local single size=1 =0; Sum_TargetChain_ObjectDx_4 local single size=1 =0; TargetChain_ObjectDx_1 local single size=80 =255; TargetChain_ObjectDx_2 local single size=80 =255; TargetChain_ObjectDx_3 local single size=80 =255; TargetChain_ObjectDx_4 local single size=80 =255; TargetChain_ObjectDx_Average_1 local single size=1 =255; TargetChain_ObjectDx_Average_2 local single size=1 =255; TargetChain_ObjectDx_Average_3 local single size=1 =255; TargetChain_ObjectDx_Average_4 local single size=1 =255; TargetChain_ObjectNum_1 local uint8 size=1 =0; TargetChain_ObjectNum_2 local uint8 size=1 =0; TargetChain_ObjectNum_3 local uint8 size=1 =0; TargetChain_ObjectNum_4 local uint8 size=1 =0; TargetChain_ObjectDx_Average output single size=80; TargetChain_ObjectDy_Average output single size=80; TargetChainPart output uint8 size=80 =0

== stateflow chart PubIfDecisionTOS_MDL/TOS_20201112/TOS_2012080320/PP1128/AAT-AdditionalAttributes/RoadEdge/RE_2020_12_07/RoadEdge_V2/RoadEdgeGroupChain/EgoLeft_RoadEdgeGroupChainInfo ==
  state REGroupChainNumCal [function]
    note: 给边界组链编号
    (default) -> (junction 181)
    (junction 181) -> (junction 190) [order 1] : [i == uint8(0)]
        | %Dx最近的目标是边界组链开始元素
    (junction 181) -> (junction 133) [order 2]
    (junction 190) -> (junction 195)
    (junction 195) -> (junction 185) [order 1] : [GroupChainStartIndex[i] != uint8(0)]
    (junction 195) -> (junction 192) [order 2] : {
        | GroupChainIndex[i] = uint8(0);
        | }
    (junction 185) -> (junction 188) : {
        | GroupChainIndex[i] = GroupChainNum;
        |  GroupChainNum = GroupChainNum + uint8(1);
        | }
    (junction 133) -> (junction 134) [order 1] : [(GroupChainStartIndex[i-uint8(1)] == uint8(0)&&...
        | GroupChainStartIndex[i] != uint8(0))||...
        | (GroupChainStartIndex[i-uint8(1)] != uint8(0)&&...
        | GroupChainStartIndex[i] != uint8(0)&&...
        | GroupChainStartIndex[i] != GroupChainStartIndex[i-uint8(1)])]
        | %边界组链开始元素
    (junction 133) -> (junction 135) [order 2]
    (junction 134) -> (junction 139) : {
        | GroupChainIndex[i] = GroupChainNum;
        |  GroupChainNum = GroupChainNum + uint8(1);
        | }
    (junction 135) -> (junction 136) [order 1] : [GroupChainStartIndex[i] != uint8(0)&&...
        | GroupChainStartIndex[i] == GroupChainStartIndex[i-uint8(1)]]
        | %边界组链剩余元素
    (junction 135) -> (junction 137) [order 2] : {
        | GroupChainIndex[i] = uint8(0);
        | }
    (junction 136) -> (junction 138) : {
        | GroupChainIndex[i] = GroupChainIndex[i-uint8(1)];
        | }
    (junction 138) -> (junction 137)
    (junction 139) -> (junction 138)
    (junction 192) -> (junction 139)
    (junction 188) -> (junction 192)
    (junction 137) -> (junction 140)
  state REGroupChainElementNumCal [function]
    (default) -> (junction 198)
    (junction 198) -> (junction 197) [order 1] : [i > uint8(1)]
    (junction 198) -> (junction 201) [order 2] : {
        | GroupChainElementNum[i] = uint8(0);
        | }
    (junction 197) -> (junction 169)
    (junction 169) -> (junction 170) [order 1] : [(GroupChainStartIndex[i-uint8(1)] != uint8(0)&&...
        | GroupChainStartIndex[i] == uint8(0))||...
        | (GroupChainStartIndex[i-uint8(1)] != uint8(0)&&...
        | GroupChainStartIndex[i] != GroupChainStartIndex[i-uint8(1)])]
        | %[i-uint8(1)]为目标链结束元素
    (junction 169) -> (junction 171) [order 2] : {
        | GroupChainElementNum[i-uint8(1)] = uint8(0);
        | }
    (junction 170) -> (junction 172) : {
        | GroupChainElementNum[i-uint8(1)] = GroupChainElementCounter[i-uint8(1)] ;
        | }
    (junction 171) -> (junction 201)
    (junction 172) -> (junction 171)
    (junction 201) -> (junction 173)
    (junction 173) -> (junction 237) [order 1] : [i > uint8(2)&&GroupChainElementNum[i-uint8(1)]  != uint8(0)]
        | %边界组链结束元素，从第3个目标开始判断，[i]目标为边界组链结束元素
    (junction 173) -> (junction 240) [order 2]
    (junction 237) -> (junction 239) : {
        | j = uint8(1);
        | }
    (junction 239) -> (junction 235) [order 1] : [ j <= GroupChainElementNum[i-uint8(1)] ]
    (junction 231) -> (junction 239) : {
        | j = j+uint8(1);
        | }
    (junction 239) -> (junction 233) [order 2]
    (junction 235) -> (junction 231) : {
        | GroupChainElementNum[i-j] = GroupChainElementNum[i-uint8(1)];
        | }
        | %同一目标链上所有元素标记目标链的元素个数
    (junction 233) -> (junction 240)
    (junction 240) -> (junction 242)
  (default) -> (junction 2) : {
      | i = uint8(0);
      | GroupChainNum=uint8(1);
      | GroupChainIndex = C_TOS_RE_80Uint8Default_Val;
      | GroupChainElementNum = C_TOS_RE_80Uint8Default_Val;
      | }
      | %从第1个目标开始
  (junction 2) -> (junction 3) [order 1] : [(RE_StillObjectSortIndex[i] ~= C_TOS_StillObjSortInvalidIndex_Val||...
      | (i > uint8(0)&&RE_StillObjectSortIndex[i-uint8(1)] ~= C_TOS_StillObjSortInvalidIndex_Val))&&...
      | i <= uint8(79)]
      | %循环到有效目标的下一个目标，保证找到边界组链的结束元素
  (junction 116) -> (junction 2) : {
      | i = i+uint8(1);
      | }
  (junction 2) -> (junction 5) [order 2]
  (junction 3) -> (junction 118) : {
      | REGroupChainNumCal();
      | }
  (junction 118) -> (junction 116) : {
      | REGroupChainElementNumCal();
      | }
  (junction 5) -> (junction 10)
  data: GroupChainIndex output uint8 size=80; C_TOS_StillObjSortInvalidIndex_Val parameter; RE_StillObjectSortIndex input size=80; i local uint8 size=1; GroupChainElementCounter input uint8 size=80; GroupChainStartIndex input uint8 size=80; GroupChainElementNum output uint8 size=80; GroupChainNum local uint8 size=1; C_TOS_RE_80Uint8Default_Val parameter; j local uint8 size=1
